simulink model "uz_ParameterID"  (R2021a)
settings: Solver=FixedStepDiscrete  StartTime=0.0  StopTime=160  FixedStep=0.000005  RelTol=1e-3  EnableMultiTasking=on
model workspace (MATLAB code in the model file):
  | cmdLim = Simulink.Parameter;
  | cmdLim.Value = 15;
  | cmdLim.Description = 'Limit for controlling the maximum surface command angle.';
  | cmdLim.Min = 0;
  | cmdLim.Max = 90;
  | cmdLim.DocUnits = 'deg';
  | 
  | dispGain = Simulink.Parameter;
  | dispGain.Value = 0.75;
  | dispGain.Description = 'Gain applied to the displacement error.';
  | dispGain.Min = 0;
  | dispGain.Max = [];
  | dispGain.DocUnits = 'deg/sec/deg';
  | 
  | dispLim = Simulink.Parameter;
  | dispLim.Value = 30;
  | dispLim.Description = 'Limit for controlling the maximum commanded angle.';
  | dispLim.Min = 0;
  | dispLim.Max = 180;
  | dispLim.DocUnits = 'deg';
  | 
  | intGain = Simulink.Parameter;
  | intGain.Value = 0.5;
  | intGain.Description = 'Gain applied to the integral error.';
  | intGain.Min = 0;
  | intGain.Max = [];
  | intGain.DocUnits = 'deg/sec/deg/sec';
  | 
  | intLim = Simulink.Parameter;
  | intLim.Value = 5;
  | intLim.Description = 'Limit for controlling the maximum commanded angle.';
  | intLim.Min = 0;
  | intLim.Max = 90;
  | intLim.DocUnits = 'deg';
  | 
  | rateGain = Simulink.Parameter;
  | rateGain.Value = 2;
  | rateGain.Description = 'Gain applied to the rate error.';
  | rateGain.Min = 0;
  | rateGain.Max = [];
  | rateGain.DocUnits = 'deg/deg/sec';
  | 
  | rateLim = Simulink.Parameter;
  | rateLim.Value = 6;
  | rateLim.Description = 'Limit for controlling the maximum commanded angle.';
  | rateLim.Min = 0;
  | rateLim.Max = 180;
  | rateLim.DocUnits = 'deg/sec';
  | 
  | hdgGain = Simulink.Parameter;
  | hdgGain.Value = 0.015;
values from neighbouring files (symbols this model uses):
  d_d_TMS = 0.005    [Parameter_Init_Buehler_201.m]
  d_f_hardware = 200000    [Parameter_Init_Buehler_201.m]
  d_f_states = 20000    [Parameter_Init_Buehler_201.m]
  d_i_max = 15    [Parameter_Init_Buehler_201.m]
  d_i_min = -d_i_max    (= -15)    [Parameter_Init_Buehler_201.m]
  d_I_n = 8    [Parameter_Init_Buehler_201.m]
  d_J_Coupling_M_E = 2e-6    (= 2e-06)    [Parameter_Init_Buehler_201.m]
  d_J_Coupling_M_Ms = 2e-20    [Parameter_Init_Buehler_201.m]
  d_J_Ms_L = d_J_Ms_M    (= 1.26363648e-05)    [Parameter_Init_Buehler_201.m]
  d_J_Ms_M = 0.5*0.5*((0.5*d_d_Ms)^4)*3.14*d_l_Ms*d_rho_Ms    (= 1.26363648e-05)    [Parameter_Init_Buehler_201.m]
  d_Ki_id = 162.47    [Parameter_Init_Buehler_201.m]
  d_Ki_iq = 162.47    [Parameter_Init_Buehler_201.m]
  d_Ki_n = 1.982    [Parameter_Init_Buehler_201.m]
  d_Kp_id = 0.369    [Parameter_Init_Buehler_201.m]
  d_Kp_iq = 0.369    [Parameter_Init_Buehler_201.m]
  d_Kp_n = 0.198    [Parameter_Init_Buehler_201.m]
  d_L_d = 0.00031    [Parameter_Init_Buehler_201.m]
  d_L_q = 0.00033    [Parameter_Init_Buehler_201.m]
  d_n_n = 3200    [Parameter_Init_Buehler_201.m]
  d_p = 4    [Parameter_Init_Buehler_201.m]
  d_psi_pm = 0.0075    [Parameter_Init_Buehler_201.m]
  d_R_ph = d_R_ph_ph/2    (= 0.089)    [Parameter_Init_Buehler_201.m]
  d_y_max = 10    [Parameter_Init_Buehler_201.m]
  d_y_min = -d_y_max    (= -10)    [Parameter_Init_Buehler_201.m]
undefined symbols (not defined in the file or in its folder): i_dq, i_dq_ref, n_ref, V_abc, v_dq
libraries: fl_lib x47, nesl_utility x30, ee_lib x18, simulink x8, spsabctodq0Lib x2, spsdq0toabcLib x1, spsTriangleGeneratorLib x1
(part 4 of 4)

== system uz_ParameterID/Hardware/Switch f. TMS/closed ==
  Input : PMIOPort  Side=Left
  output : PMIOPort  Port=2  Side=Right
  connections:
  output/RConn1 -- Input/RConn1

== system uz_ParameterID/Hardware/Switch f. TMS/open ==
  Rotational Free End : fl_lib/Mechanical/Rotational Elements/Rotational Free End  w_specify=off  w_priority=None  w=0 rad/s  w_nominal_specify=off  w_nominal_unit=rad/s  w_nominal_value=1
      settings: SourceProductBaseCode=SS
  Rotational Free End1 : fl_lib/Mechanical/Rotational Elements/Rotational Free End  w_specify=off  w_priority=None  w=0 rad/s  w_nominal_specify=off  w_nominal_unit=rad/s  w_nominal_value=1
      settings: SourceProductBaseCode=SS
  Input : PMIOPort  Side=Left
  output : PMIOPort  Port=2  Side=Right
  connections:
  Rotational Free End1/LConn1 -- output/RConn1
  Input/RConn1 -- Rotational Free End/LConn1

== system uz_ParameterID/Hardware/coupling m. shaft/Inertia ==
  Trägheitsmoment3 : fl_lib/Mechanical/Rotational Elements/Inertia  Commented=on  inertia=d_J_Coupling_M_Ms kg*m^2  num_ports=foundation.enum.numPorts2.one  w_specify=off  w_priority=High  w=0 rad/s  w_nominal_specify=off  w_nominal_unit=rad/s  w_nominal_value=1  t_specify=off  t_priority=None  t=0 N*m  t_nominal_specify=off  t_nominal_unit=N*m  t_nominal_value=1
      settings: AttributesFormatString=J in [%<inertia_unit>]
  Input : PMIOPort  Side=Left
  output : PMIOPort  Port=2  Side=Right
  connections:
  Input/RConn1 -- Trägheitsmoment3/LConn1 -- output/RConn1

== system uz_ParameterID/Hardware/coupling m. shaft/Spring Damper System ==
  Rotational Spring : fl_lib/Mechanical/Rotational Elements/Rotational Spring  spr_rate=d_c_Coupling_M_Ms N*m/rad  w_specify=off  w_priority=None  w=0 rad/s  w_nominal_specify=off  w_nominal_unit=rad/s  w_nominal_value=1  t_specify=off  t_priority=None  t=0 N*m  t_nominal_specify=off  t_nominal_unit=N*m  t_nominal_value=1  phi_specify=off  phi_priority=High  phi=0 rad  phi_nominal_specify=off  phi_nominal_unit=rad  phi_nominal_value=1
  Trägheitsmoment1 : fl_lib/Mechanical/Rotational Elements/Inertia  inertia=d_J_Coupling_M_Ms/2 kg*m^2  num_ports=foundation.enum.numPorts2.one  w_specify=off  w_priority=High  w=0 rad/s  w_nominal_specify=off  w_nominal_unit=rad/s  w_nominal_value=1  t_specify=off  t_priority=None  t=0 N*m  t_nominal_specify=off  t_nominal_unit=N*m  t_nominal_value=1
      settings: AttributesFormatString=J in [%<inertia_unit>]
  Trägheitsmoment3 : fl_lib/Mechanical/Rotational Elements/Inertia  inertia=d_J_Coupling_M_Ms/2 kg*m^2  num_ports=foundation.enum.numPorts2.one  w_specify=off  w_priority=High  w=0 rad/s  w_nominal_specify=off  w_nominal_unit=rad/s  w_nominal_value=1  t_specify=off  t_priority=None  t=0 N*m  t_nominal_specify=off  t_nominal_unit=N*m  t_nominal_value=1
      settings: AttributesFormatString=J in [%<inertia_unit>]
  dm : fl_lib/Mechanical/Rotational Elements/Rotational Damper  Commented=on  D=0 N*m/(rad/s)  w_specify=off  w_priority=None  w=0 rad/s  w_nominal_specify=off  w_nominal_unit=rad/s  w_nominal_value=1  t_specify=off  t_priority=None  t=0 N*m  t_nominal_specify=off  t_nominal_unit=N*m  t_nominal_value=1
  Input : PMIOPort  Side=Left
  output : PMIOPort  Port=2  Side=Right
  connections:
  Rotational Spring/LConn1 -- dm/LConn1 -- Input/RConn1 -- Trägheitsmoment3/LConn1
  Trägheitsmoment1/LConn1 -- Rotational Spring/RConn1 -- dm/RConn1 -- output/RConn1

== system uz_ParameterID/FOC/uz_FOC_Current/id-PI-Controller with anti wind-up/Clamping circuit ==
  preSat : Inport  DisableCoverage=on  OutDataTypeStr=single
  preIntegrator : Inport  DisableCoverage=on  Port=2
  AND : Logic  DisableCoverage=on
  DataTypeConv1 : DataTypeConversion  DisableCoverage=on  OutDataTypeStr=int8  SaturateOnIntegerOverflow=on  RndMeth=Zero  LockScale=on
  DataTypeConv2 : DataTypeConversion  DisableCoverage=on  OutDataTypeStr=int8  SaturateOnIntegerOverflow=on  RndMeth=Zero  LockScale=on
  DeadZone : DeadZone  DisableCoverage=on  LowerValue=d_y_min  UpperValue=d_y_max  SaturateOnIntegerOverflow=on
  Equal : RelationalOperator  DisableCoverage=on  Operator===  RndMeth=Nearest  InputSameDT=on
  NotEqual : RelationalOperator  DisableCoverage=on  Operator=~=  RndMeth=Nearest  InputSameDT=on
  SignDeltaU : Signum  DisableCoverage=on
  SignPreIntegrator : Signum  DisableCoverage=on
  ZeroGain : Gain  DisableCoverage=on  Gain=0  ParamDataTypeStr=double  OutDataTypeStr=single  SaturateOnIntegerOverflow=on
  Clamp : Outport  DisableCoverage=on  VectorParamsAs1DForOutWhenUnconnected=off
  wires:
  preSat/1 -> ZeroGain/1, DeadZone/1
  preIntegrator/1 -> SignPreIntegrator/1
  ZeroGain/1 -> NotEqual/1
  DeadZone/1 -> NotEqual/2, SignDeltaU/1
  SignDeltaU/1 -> DataTypeConv1/1
  DataTypeConv1/1 -> Equal/1
  SignPreIntegrator/1 -> DataTypeConv2/1
  DataTypeConv2/1 -> Equal/2
  NotEqual/1 -> AND/1
  Equal/1 -> AND/2
  AND/1 -> Clamp/1

== system uz_ParameterID/FOC/uz_FOC_Current/iq-PI-Controller with anti wind-up/Clamping circuit ==
  preSat : Inport  DisableCoverage=on  OutDataTypeStr=single
  preIntegrator : Inport  DisableCoverage=on  Port=2
  AND : Logic  DisableCoverage=on
  DataTypeConv1 : DataTypeConversion  DisableCoverage=on  OutDataTypeStr=int8  SaturateOnIntegerOverflow=on  RndMeth=Zero  LockScale=on
  DataTypeConv2 : DataTypeConversion  DisableCoverage=on  OutDataTypeStr=int8  SaturateOnIntegerOverflow=on  RndMeth=Zero  LockScale=on
  DeadZone : DeadZone  DisableCoverage=on  LowerValue=d_y_min  UpperValue=d_y_max  SaturateOnIntegerOverflow=on
  Equal : RelationalOperator  DisableCoverage=on  Operator===  RndMeth=Nearest  InputSameDT=on
  NotEqual : RelationalOperator  DisableCoverage=on  Operator=~=  RndMeth=Nearest  InputSameDT=on
  SignDeltaU : Signum  DisableCoverage=on
  SignPreIntegrator : Signum  DisableCoverage=on
  ZeroGain : Gain  DisableCoverage=on  Gain=0  ParamDataTypeStr=double  OutDataTypeStr=single  SaturateOnIntegerOverflow=on
  Clamp : Outport  DisableCoverage=on  VectorParamsAs1DForOutWhenUnconnected=off
  wires:
  preSat/1 -> ZeroGain/1, DeadZone/1
  preIntegrator/1 -> SignPreIntegrator/1
  ZeroGain/1 -> NotEqual/1
  DeadZone/1 -> NotEqual/2, SignDeltaU/1
  SignDeltaU/1 -> DataTypeConv1/1
  DataTypeConv1/1 -> Equal/1
  SignPreIntegrator/1 -> DataTypeConv2/1
  DataTypeConv2/1 -> Equal/2
  NotEqual/1 -> AND/1
  Equal/1 -> AND/2
  AND/1 -> Clamp/1

== system uz_ParameterID/FOC/uz_FOC_Speed/omega-PI-Controller with anti wind-up/Clamping circuit ==
  preSat : Inport  DisableCoverage=on  OutDataTypeStr=single
  preIntegrator : Inport  DisableCoverage=on  Port=2
  AND : Logic  DisableCoverage=on
  DataTypeConv1 : DataTypeConversion  DisableCoverage=on  OutDataTypeStr=int8  SaturateOnIntegerOverflow=on  RndMeth=Zero  LockScale=on
  DataTypeConv2 : DataTypeConversion  DisableCoverage=on  OutDataTypeStr=int8  SaturateOnIntegerOverflow=on  RndMeth=Zero  LockScale=on
  DeadZone : DeadZone  DisableCoverage=on  LowerValue=d_i_min  UpperValue=d_i_max  SaturateOnIntegerOverflow=on
  Equal : RelationalOperator  DisableCoverage=on  Operator===  RndMeth=Nearest  InputSameDT=on
  NotEqual : RelationalOperator  DisableCoverage=on  Operator=~=  RndMeth=Nearest  InputSameDT=on
  SignDeltaU : Signum  DisableCoverage=on
  SignPreIntegrator : Signum  DisableCoverage=on
  ZeroGain : Gain  DisableCoverage=on  Gain=0  ParamDataTypeStr=double  OutDataTypeStr=single  SaturateOnIntegerOverflow=on
  Clamp : Outport  DisableCoverage=on  VectorParamsAs1DForOutWhenUnconnected=off
  wires:
  preSat/1 -> ZeroGain/1, DeadZone/1
  preIntegrator/1 -> SignPreIntegrator/1
  ZeroGain/1 -> NotEqual/1
  DeadZone/1 -> NotEqual/2, SignDeltaU/1
  SignDeltaU/1 -> DataTypeConv1/1
  DataTypeConv1/1 -> Equal/1
  SignPreIntegrator/1 -> DataTypeConv2/1
  DataTypeConv2/1 -> Equal/2
  NotEqual/1 -> AND/1
  Equal/1 -> AND/2
  AND/1 -> Clamp/1

== matlab function uz_ParameterID/Hardware/12bit ADC1 ==
  data: u input; y output
function y = fcn(u)
%#codegen

y = u*2048/5;

== matlab function uz_ParameterID/Hardware/12bit ADC ==
  data: u input; y output
function y = fcn(u)
%#codegen

y = u*2048/5;

== matlab function uz_ParameterID/Hardware/12bit ADC2 ==
  data: u input; y output
function y = fcn(u)
%#codegen

y = u*2048/5;

== matlab function uz_ParameterID/FOC/Busselector ==
  data: ControlFlags input Bus: uz_ParaID_ControlFlags_t; FOC_state_outputs output Bus: uz_ParaID_Controller_Parameters_output_t; ElectricalID_FOC_input input Bus: uz_ParaID_Controller_Parameters_output_t; FrictionID_FOC_input input Bus: uz_ParaID_Controller_Parameters_output_t; FluxMapID_FOC_input input Bus: uz_ParaID_Controller_Parameters_output_t; TwoMassID_FOC_input input Bus: uz_ParaID_Controller_Parameters_output_t; FOCControl_input input Bus: uz_ParaID_Controller_Parameters_output_t
function FOC_state_outputs = fcn(ControlFlags,ElectricalID_FOC_input,....
    FrictionID_FOC_input,FluxMapID_FOC_input,TwoMassID_FOC_input,FOCControl_input)

switch ControlFlags.transNr
    case 0
        if(ControlFlags.finished_all_Offline_states==1)
            FOC_state_outputs           = FOCControl_input;
        else
        FOC_state_outputs.i_dq_ref.d          = single(0);
        FOC_state_outputs.i_dq_ref.q          = single(0);
        FOC_state_outputs.i_dq_ref.zero       = single(0);
        FOC_state_outputs.activeState         = uint16(0);
        FOC_state_outputs.n_ref_FOC           = single(0);
        FOC_state_outputs.enableFOC_speed     = boolean(0);
        FOC_state_outputs.enableFOC_current   = boolean(0);
        FOC_state_outputs.resetIntegrator     = boolean(0);
        FOC_state_outputs.Kp_id_out           = single(0);
        FOC_state_outputs.Kp_iq_out           = single(0);
        FOC_state_outputs.Kp_n_out            = single(0);
        FOC_state_outputs.Ki_id_out           = single(0);
        FOC_state_outputs.Ki_iq_out           = single(0);
        FOC_state_outputs.Ki_n_out            = single(0);
        end
    case 1
        FOC_state_outputs           = ElectricalID_FOC_input;
    case 2
        FOC_state_outputs           = TwoMassID_FOC_input;
    case 3
        FOC_state_outputs           = FrictionID_FOC_input;
    case 4
        FOC_state_outputs           = FluxMapID_FOC_input;
    otherwise
        FOC_state_outputs.i_dq_ref.d          = single(0);
        FOC_state_outputs.i_dq_ref.q          = single(0);
        FOC_state_outputs.i_dq_ref.zero       = single(0);
        FOC_state_outputs.activeState         = uint16(0);
        FOC_state_outputs.n_ref_FOC           = single(0);
        FOC_state_outputs.enableFOC_speed     = boolean(0);
        FOC_state_outputs.enableFOC_current   = boolean(0);
        FOC_state_outputs.resetIntegrator     = boolean(0);
        FOC_state_outputs.Kp_id_out           = single(0);
        FOC_state_outputs.Kp_iq_out           = single(0);
        FOC_state_outputs.Kp_n_out            = single(0);
        FOC_state_outputs.Ki_id_out           = single(0);
        FOC_state_outputs.Ki_iq_out           = single(0);
        FOC_state_outputs.Ki_n_out            = single(0);
end
end

== stateflow chart uz_ParameterID/ControlState ==
  settings: updateMethod=DISCRETE  sampleTime=1/d_f_states
  note: ControlState
  state ControlState
    entry:
    during:
    GlobalConfig_out.Reset = GlobalConfig_in.Reset;
    GlobalConfig_out.ACCEPT = GlobalConfig_in.ACCEPT;
    GlobalConfig_out.enableParameterID = GlobalConfig_in.enableParameterID;
    GlobalConfig_out.ElectricalID = GlobalConfig_in.ElectricalID;
    GlobalConfig_out.FrictionID = GlobalConfig_in.FrictionID
    GlobalConfig_out.TwoMassID = GlobalConfig_in.TwoMassID;
    GlobalConfig_out.FluxMapID = GlobalConfig_in.FluxMapID;
    GlobalConfig_out.OnlineID = GlobalConfig_in.OnlineID;
    GlobalConfig_out.sampleTimeISR = GlobalConfig_in.sampleTimeISR;
    state decideMotorID
      entry:
      during:
      if (GlobalConfig_in.ACCEPT == 1)
      decideIDstates;
      end
      if(ControlFlags.finished_all_Offline_states == 1 && GlobalConfig_in.OnlineID==1 && enteredOnlineID==0)
      ControlFlags.enableOnlineID=boolean(1);
      elseif (ControlFlags.finished_all_Offline_states == 1 && GlobalConfig_in.OnlineID==0 && enteredOnlineID==1)
      ControlFlags.enableOnlineID=boolean(0);
      end
      exit:
    state activateFrictionID
      entry:
      ControlFlags.startFrictionID=boolean(1);
      during:
      exit:
    state activateFluxMapID
      entry:
      ControlFlags.startFluxMapID=boolean(1);
      during:
      exit:
    state activateTwoMassID
      entry:
      ControlFlags.startTwoMassID=boolean(1);
      during:
      exit:
    state activateElectricalID
      entry:
      ControlFlags.startElectricalID=boolean(1);
      during:
      exit:
    state duringElectricalID
      entry:
      ControlFlags.startElectricalID=boolean(0);
      during:
      GlobalConfig_out.PMSM_config.Ld_Henry=ElectricalID_output.PMSM_parameters.Ld_Henry;
      GlobalConfig_out.PMSM_config.Lq_Henry=ElectricalID_output.PMSM_parameters.Lq_Henry;
      GlobalConfig_out.PMSM_config.R_ph_Ohm=ElectricalID_output.PMSM_parameters.R_ph_Ohm;
      GlobalConfig_out.PMSM_config.Psi_PM_Vs=ElectricalID_output.PMSM_parameters.Psi_PM_Vs;
      GlobalConfig_out.PMSM_config.polePairs=ElectricalID_output.PMSM_parameters.polePairs;
      GlobalConfig_out.PMSM_config.J_kg_m_squared=....
      ElectricalID_output.PMSM_parameters.J_kg_m_squared;
      GlobalConfig_out.Kp_id=ElectricalID_FOC_output.Kp_id_out;
      GlobalConfig_out.Kp_iq=ElectricalID_FOC_output.Kp_iq_out;
      GlobalConfig_out.Kp_n=ElectricalID_FOC_output.Kp_n_out;
      GlobalConfig_out.Ki_id=ElectricalID_FOC_output.Ki_id_out;
      GlobalConfig_out.Ki_iq=ElectricalID_FOC_output.Ki_iq_out;
      GlobalConfig_out.Ki_n=ElectricalID_FOC_output.Ki_n_out;
      exit:
    state duringTwoMassID
      entry:
      ControlFlags.startTwoMassID=boolean(0);
      during:
      exit:
    state duringFrictionID
      entry:
      ControlFlags.startFrictionID=boolean(0);
      during:
      exit:
    state duringFluxMapID
      entry:
      ControlFlags.startFluxMapID=boolean(0);
      during:
      exit:
    state finishedFrictionID
      entry:
      finishedFrictionID_loc=uint16(2);
      during:
      exit:
      ControlFlags.transNr=uint16(0);
    state finishedFluxMapID
      entry:
      finishedFluxMapID_loc=uint16(2);
      during:
      exit:
      ControlFlags.transNr=uint16(0);
    state finishedTwoMassID
      entry:
      finishedTwoMassID_loc=uint16(2);
      during:
      exit:
      ControlFlags.transNr=uint16(0);
    state finishedElectricalID
      entry:
      finishedElectricalID_loc=uint16(2);
      during:
      exit:
      ControlFlags.transNr=uint16(0);
    (default) -> decideMotorID
    decideMotorID -> activateElectricalID [order 1] : [ControlFlags.transNr==1 && finishedElectricalID_loc==0]
    activateElectricalID -> decideMotorID [order 2] : [GlobalConfig_in.ElectricalID==0]
        | {ControlFlags.transNr = 0}
    duringElectricalID -> decideMotorID [order 2] : [GlobalConfig_in.ElectricalID==0]
        | {ControlFlags.transNr = 0}
    finishedElectricalID -> decideMotorID
    finishedTwoMassID -> decideMotorID
    decideMotorID -> activateTwoMassID [order 3] : [ControlFlags.transNr==2 && finishedTwoMassID_loc==0]
    activateTwoMassID -> decideMotorID [order 2] : [GlobalConfig_in.TwoMassID==0]
        | {ControlFlags.transNr = 0}
    duringTwoMassID -> decideMotorID [order 2] : [GlobalConfig_in.TwoMassID==0]
        | {ControlFlags.transNr = 0}
    finishedFrictionID -> decideMotorID
    decideMotorID -> activateFrictionID [order 4] : [ControlFlags.transNr==3 && finishedFrictionID_loc==0]
    activateFrictionID -> decideMotorID [order 2] : [GlobalConfig_in.FrictionID==0]
        | {ControlFlags.transNr = 0}
    duringFrictionID -> decideMotorID [order 2] : [GlobalConfig_in.FrictionID==0]
        | {ControlFlags.transNr = 0}
    finishedFluxMapID -> decideMotorID
    decideMotorID -> activateFluxMapID [order 2] : [ControlFlags.transNr==4 && finishedFluxMapID_loc==0]
    activateFluxMapID -> decideMotorID [order 2] : [GlobalConfig_in.FluxMapID==0]
        | {ControlFlags.transNr = 0}
    duringFluxMapID -> decideMotorID [order 2] : [GlobalConfig_in.FluxMapID==0]
        | {ControlFlags.transNr = 0}
    activateElectricalID -> duringElectricalID [order 1] : [enteredElectricalID==1]
    activateTwoMassID -> duringTwoMassID [order 1] : [enteredTwoMassID==1]
    activateFrictionID -> duringFrictionID [order 1] : [enteredFrictionID==1]
    activateFluxMapID -> duringFluxMapID [order 1] : [enteredFluxMapID==1]
    duringTwoMassID -> finishedTwoMassID [order 1] : [finishedTwoMassID==1]
    duringFrictionID -> finishedFrictionID [order 1] : [finishedFrictionID==1]
    duringFluxMapID -> finishedFluxMapID [order 1] : [finishedFluxMapID==1]
    duringElectricalID -> finishedElectricalID [order 1] : [finishedElectricalID==1]
  state Waiting
    entry:
    initParams;
    %wait for activation of
    %FrictionID
    %donothing
  note: ---
  Waiting -> ControlState [order 1] : [GlobalConfig_in.enableParameterID==1 && ....
      | GlobalConfig_in.Reset==0]
  (default) -> Waiting
  ControlState -> Waiting : [GlobalConfig_in.Reset==1 ||....
      |  GlobalConfig_in.enableParameterID==0]
  Waiting -> Waiting [order 2] : [GlobalConfig_in.Reset==1]
  data: finishedFrictionID input boolean; finishedElectricalID input boolean; finishedTwoMassID input boolean; finishedFluxMapID input boolean; enteredFrictionID input boolean; enteredFluxMapID input boolean; enteredTwoMassID input boolean; enteredElectricalID input boolean; ElectricalID_output input Bus: uz_ParaID_ElectricalID_output_t; finishedElectricalID_loc local; finishedFrictionID_loc local; finishedTwoMassID_loc local; finishedFluxMapID_loc local; ElectricalID_FOC_output input Bus: uz_ParaID_Controller_Parameters_output_t; GlobalConfig_in input Bus: uz_ParaID_GlobalConfig_t; GlobalConfig_out output Bus: uz_ParaID_GlobalConfig_t; ControlFlags output Bus: uz_ParaID_ControlFlags_t; enteredOnlineID input
  function decideIDstates:
    | function decideIDstates
    | %If the specific Identification Part is not selected (==0), treat it, as if
    | %it has finished
    | if(GlobalConfig_in.ElectricalID==0)
    |     finishedElectricalID_loc=uint16(1);
    | elseif(finishedElectricalID==1)
    |     finishedElectricalID_loc=uint16(2);
    | end
    | 
    | if(GlobalConfig_in.FrictionID==0)
    |     finishedFrictionID_loc=uint16(1);
    | elseif(finishedFrictionID==1)
    |      finishedFrictionID_loc=uint16(2);
    | end
    | 
    | if(GlobalConfig_in.TwoMassID==0)
    |     finishedTwoMassID_loc=uint16(1);
    | elseif(finishedTwoMassID==1)
    |     finishedTwoMassID_loc=uint16(2);
    | end
    | 
    | if(GlobalConfig_in.FluxMapID==0)
    |     finishedFluxMapID_loc=uint16(1);
    | elseif(finishedFluxMapID==1)
    |     finishedFluxMapID_loc=uint16(2);    
    | end
    | 
    | if(ControlFlags.finished_all_Offline_states == 0)
    |     %Determine path through the ElectricalID-Stateflows
    |     if(GlobalConfig_in.ElectricalID==1 && enteredElectricalID==0 && finishedElectricalID_loc~=2 && finishedElectricalID==0)
    |             ControlFlags.transNr=uint16(1);
    |             finishedElectricalID_loc = uint16(0);
    |     end
    | 
    |     %Determine path through the TwoMassID-Stateflows
    |     if(GlobalConfig_in.TwoMassID==1 && enteredTwoMassID==0 && finishedElectricalID_loc~=0 && finishedTwoMassID_loc~=2 && finishedTwoMassID==0)
    |             ControlFlags.transNr=uint16(2);
    |             finishedTwoMassID_loc = uint16(0);
    |     end
    |     
    |     %Determine path through the FrictionID-Stateflows
    |     if(GlobalConfig_in.FrictionID==1 && enteredFrictionID==0 && finishedElectricalID_loc~=0....
    |        && finishedTwoMassID_loc~=0 && finishedFrictionID_loc~=2 && finishedFrictionID==0)
    |            ControlFlags.transNr=uint16(3);
    |            finishedFrictionID_loc = uint16(0);
    |     end
    | 
    |     %Determine path through the FluxMapID-Stateflows
    |     if(GlobalConfig_in.FluxMapID==1 && enteredFluxMapID==0 && finishedElectricalID_loc~=0....
    |       && finishedTwoMassID_loc~=0 && finishedFrictionID_loc~=0 && finishedFluxMapID_loc~=2 && finishedFluxMapID==0)
    |             ControlFlags.transNr=uint16(4);
    |             finishedFluxMapID_loc = uint16(0);
    |     end
    | end
    | 
    | if(finishedElectricalID_loc~=0 && finishedTwoMassID_loc~=0 && ....
    |         finishedFrictionID_loc~=0 && finishedFluxMapID_loc~=0)
    |     ControlFlags.finished_all_Offline_states = boolean(1);
    | end
    | 
    | end
  function initParams:
    | function initParams
    | %Initialize Variables
    | finishedElectricalID_loc=uint16(0);
    | finishedFrictionID_loc=uint16(0);
    | finishedTwoMassID_loc=uint16(0);
    | finishedFluxMapID_loc=uint16(0);
    | 
    | %Initialize Outputs
    | ControlFlags.startFrictionID             = boolean(0);
    | ControlFlags.startElectricalID           = boolean(0);
    | ControlFlags.startTwoMassID              = boolean(0);
    | ControlFlags.startFluxMapID              = boolean(0);
    | GlobalConfig_out                         = GlobalConfig_in;
    | ControlFlags.enableOnlineID              = boolean(0);
    | ControlFlags.transNr                     = uint16(0);
    | ControlFlags.finished_all_Offline_states = boolean(0);
    | end

== matlab function uz_ParameterID/InterpMeshGrid ==
  data: FluxMapData output Bus: uz_ParaID_FluxMapsData_t; psi_array_in input; i_rat input; OnlineID_input input
function FluxMapData = fcn(psi_array_in,i_rat,OnlineID_input)
%Author Philipp Gebhardt
% Oktober 2019

%This function is calculating the regular flux maps out of the irregular scatter data array stored in psi_array_in. The Outputs rangeX are containg the flux maps axis information which range is related to 3 times i_rat input.
%Furthermore the temperature dependency of the permanent flux is calculated if there are enough measuring values stored in the delta_psi_array. The temperature constant as well as the estimated error of permanent flux
%at reference temperature are given out on psi_temp_const and psi_temp_error outputs.  Using this temperature dependency the flux maps are updated with the permanent flux offset caused by the temperature which is given
%in on OnlineID_input.Wtemp input. 

%-----------------------------------------------------------------------------------------------------------------------------------------
%initalising Outputs
%-----------------------------------------------------------------------------------------------------------------------------------------

psi_array=zeros(6,100);
psi_array=psi_array_in;
delta_psi=zeros(100,1);

FluxMapData.psid_grid=single(zeros(20,20));
FluxMapData.psiq_grid=single(zeros(20,20));
FluxMapData.id_grid=single(zeros(20,20));
FluxMapData.iq_grid=single(zeros(20,20));
FluxMapData.range_id_Y=single(zeros(1,20));
FluxMapData.range_psid_Y=single(zeros(1,20));
FluxMapData.range_psiq_Y=single(zeros(1,20));
FluxMapData.range_psid_X=single(zeros(1,20));
FluxMapData.range_psiq_X=single(zeros(1,20));
FluxMapData.range_iq_Y=single(zeros(1,20));
FluxMapData.range_iq_X=single(zeros(1,20));
FluxMapData.range_id_X=single(zeros(1,20));
FluxMapData.psi_temp_const=single(0.000001);
FluxMapData.psi_temp_error=single(0);



range_psid_X_in=single(zeros(1,20));
range_psid_Y_in=single(zeros(1,20));
range_psiq_X_in=single(zeros(1,20));
range_psiq_Y_in=single(zeros(1,20));
range_id_X_in=single(zeros(1,20));
range_id_Y_in=single(zeros(1,20));
range_iq_X_in=single(zeros(1,20));
range_iq_Y_in=single(zeros(1,20));


%initalise range of flux maps axis
for t=single(0):single(19)
   range_psid_X_in(t+1)=-3*i_rat+t*4*i_rat/19;
   range_psid_Y_in(t+1)=-3*i_rat+t*6*i_rat/19;
   range_psiq_X_in(t+1)=-3*i_rat+t*4*i_rat/19;
   range_psiq_Y_in(t+1)=-3*i_rat+t*6*i_rat/19;
end

%Calculate flux deviation from amout of measuring values and counter sum,
%to average a big amount of measuring values 

for t=single(1):single(100)
    if (OnlineID_input.delta_psi(t,2)>5)
    delta_psi(t,1)=OnlineID_input.delta_psi(t,1)/OnlineID_input.delta_psi(t,2);
    end
end

%Calculate temperature constant with a regressionline, set second input "1"
%to resist outliers greater than 30% (relative to their neighbours)

[psi_temp_const_test,FluxMapData.psi_temp_error]=regressionline(delta_psi,1);

%check plausibility
if(psi_temp_const_test>0&&FluxMapData.psi_temp_const<10)%in mVs/°C
FluxMapData.psi_temp_const=psi_temp_const_test;
end


%correct temperature offset
 for k=single(1):single(100)
   if(psi_array(3,k)~=0)
    psi_array(5,k)=psi_array(5,k)+(psi_array(4,k)-OnlineID_input.Wtemp)*FluxMapData.psi_temp_const;
    psi_array(4,k)=OnlineID_input.Wtemp;
   end
end





%Inter- and extrapolation of the flux maps 
[FluxMapData.range_psid_X,FluxMapData.range_psid_Y,FluxMapData.psid_grid] = interpol_flux_scatter_psid ([psi_array(1,:);psi_array(2,:);psi_array(5,:);zeros(length(psi_array(1,:)))],range_psid_X_in,range_psid_Y_in);
[FluxMapData.range_psiq_X,FluxMapData.range_psiq_Y,FluxMapData.psiq_grid] = interpol_flux_scatter_psiq ([psi_array(1,:);psi_array(2,:);psi_array(6,:);zeros(length(psi_array(1,:)))],range_psiq_X_in,range_psiq_Y_in);

%initialise range of inverse flux maps axis
for t=single(0):single(19)
   range_id_X_in(t+1)=min(min(FluxMapData.psid_grid))+t*(max(max(FluxMapData.psid_grid))-min(min(FluxMapData.psid_grid)))/19;
   range_id_Y_in(t+1)=min(min(FluxMapData.psiq_grid))+t*(max(max(FluxMapData.psiq_grid))-min(min(FluxMapData.psiq_grid)))/19;
   range_iq_X_in(t+1)=min(min(FluxMapData.psid_grid))+t*(max(max(FluxMapData.psid_grid))-min(min(FluxMapData.psid_grid)))/19;
   range_iq_Y_in(t+1)=min(min(FluxMapData.psiq_grid))+t*(max(max(FluxMapData.psiq_grid))-min(min(FluxMapData.psiq_grid)))/19;
end

%Inter and extrapolate inverse flux maps
[FluxMapData.range_id_X,FluxMapData.range_id_Y,FluxMapData.id_grid] = interpol_flux_scatter_psid ([psi_array(5,:);psi_array(6,:);psi_array(1,:);zeros(length(psi_array(1,:)))],range_id_X_in,range_id_Y_in);
[FluxMapData.range_iq_X,FluxMapData.range_iq_Y,FluxMapData.iq_grid] = interpol_flux_scatter_psiq ([psi_array(5,:);psi_array(6,:);psi_array(2,:);zeros(length(psi_array(1,:)))],range_iq_X_in,range_iq_Y_in);

end

== stateflow chart uz_ParameterID/AutoRefCurrents ==
  settings: updateMethod=DISCRETE  sampleTime=1/d_f_states
  note: Philipp Gebhardt, October2019:
      |
      | Description of Control Reference Stateflow:
      |
      | This Stateflow chart is used to generate an cyclic current reference input of d- and q- current. The combinations are circularly arranged in the radius of imax_in.
      | The inputs niq and nid are the amount of measuring values in q- and d-current axis. The input speed_in is used to automatically control the sign of q-current to avoid
      | regenerative current feedback into the inverter.
  state waitState
    entry:
    %do nothing
    %wait for start
  state superstate
    entry:
    counter=single(19998);
    %counter=single(17498);
    iqcount=single(0);
    idcount=single(-AutoRefCurrentsConfig.id_points/3);
    AutoRefCurrents_output.i_dq_ref.d=single(0);
    AutoRefCurrents_output.i_dq_ref.q=single(0);
    imax=single(0);
    state stepstate
      entry:
      if(ActualValues.omega_m>0)
      imax=abs(AutoRefCurrentsConfig.max_current);
      end
      if(ActualValues.omega_m<0)
      imax=abs(AutoRefCurrentsConfig.max_current)*-1;
      end
      if((AutoRefCurrents_output.i_dq_ref.d*AutoRefCurrents_output.i_dq_ref.d+(imax*iqcount/AutoRefCurrentsConfig.iq_points)^2)^0.5<abs(imax))
      AutoRefCurrents_output.i_dq_ref.q=imax*iqcount/AutoRefCurrentsConfig.iq_points;
      else
      iqcount=single(1);
      AutoRefCurrents_output.i_dq_ref.q=imax*iqcount/AutoRefCurrentsConfig.iq_points;
      end
      if((AutoRefCurrents_output.i_dq_ref.q*AutoRefCurrents_output.i_dq_ref.q+(imax*idcount/AutoRefCurrentsConfig.id_points)^2)^0.5<abs(imax))
      AutoRefCurrents_output.i_dq_ref.d=-1*abs(imax)*idcount/AutoRefCurrentsConfig.id_points;
      else
      idcount=single(-AutoRefCurrentsConfig.id_points/3);
      AutoRefCurrents_output.i_dq_ref.d=-1*abs(imax)*idcount/AutoRefCurrentsConfig.id_points;
      end
      counter=single(0);
    state countstate
      entry:
      if(iqcount<AutoRefCurrentsConfig.iq_points)
      iqcount=iqcount+1;
      else
      iqcount=single(0);
      end
      if(idcount<AutoRefCurrentsConfig.id_points)
      idcount=idcount+1;
      else
      idcount=single(-AutoRefCurrentsConfig.id_points/3);
      end
      during:
      counter=counter+1;
    (default) -> countstate
    countstate -> stepstate : [counter==(2.0/GlobalConfig.sampleTimeISR)]
    stepstate -> countstate : [counter==0]
  (default) -> waitState
  waitState -> superstate : [AutoRefCurrentsConfig.enableCRS==1 &&....
      | AutoRefCurrentsConfig.Reset==0 &&....
      |  GlobalConfig.Reset==0 && GlobalConfig.ACCEPT==1&& ....
      | ControlFlags.finished_all_Offline_states==1]
  superstate -> waitState : [AutoRefCurrentsConfig.enableCRS==0 ||....
      |  AutoRefCurrentsConfig.Reset == 1 ||....
      | GlobalConfig.Reset==1]
      | {AutoRefCurrents_output.i_dq_ref.d=single(0);
      | AutoRefCurrents_output.i_dq_ref.q=single(0)}
  data: iqcount local; idcount local; counter local; ActualValues input Bus: uz_ParaID_ActualValues_t; imax local; GlobalConfig input Bus: uz_ParaID_GlobalConfig_t; AutoRefCurrentsConfig input Bus: uz_ParaID_AutoRefCurrentsConfig_t; AutoRefCurrents_output output Bus: uz_ParaID_AutoRefCurrents_output_t; ControlFlags input Bus: uz_ParaID_ControlFlags_t

== stateflow chart uz_ParameterID/FOC_ControlState ==
  settings: updateMethod=DISCRETE  sampleTime=1/d_f_states
  note: Control-States
  state FOC_ControlState
    entry:
    FOCControl_output.activeState = uint16(600);
    initParams;
    during:
    note: FOC current control
    state FOCcurrentControl 	%state 140
      entry:
      FOCControl_output.activeState = uint16(610);
      FOCControl_output.enableFOC_current=boolean(1);
      counter = uint32(1);
      during:
      FOCControl_output.i_dq_ref.q=GlobalConfig.i_dq_ref.q;
      FOCControl_output.i_dq_ref.d=GlobalConfig.i_dq_ref.d+i_d_Online_ref;
      exit:
      counter = uint32(1);
      FOCControl_output.enableFOC_current=boolean(0);
    state FOCdecider
      entry:
    note: FOC speed control
    note: change speed with sinusoidal trajectory in 0.2 sec
    state FOCspeed_speedChange 	%state 13.0
      entry:
      FOCControl_output.activeState = uint16(620);
      FOCControl_output.enableFOC_speed=boolean(1);
      counter = uint32(1);
      during:
      FOCControl_output.i_dq_ref.d = i_d_Online_ref+GlobalConfig.i_dq_ref.d;
      n_filt = single((single(counter)*GlobalConfig.sampleTimeISR*5)-....
      1/(2*pi)*sin(2*pi*single(counter)*GlobalConfig.sampleTimeISR*5));
      FOCControl_output.n_ref_FOC=((GlobalConfig.n_ref-n_ref_old)*n_filt)+n_ref_old;
      counter = counter + 1;
      exit:
      counter = uint32(1);
    state FOCspeed_constantSpeed 		%state 13.1
      entry:
      FOCControl_output.activeState = uint16(621);
      n_ref_old = GlobalConfig.n_ref;
      during:
      FOCControl_output.n_ref_FOC=GlobalConfig.n_ref;
      FOCControl_output.i_dq_ref.d=GlobalConfig.i_dq_ref.d +i_d_Online_ref;
      exit:
      counter = uint32(1);
      FOCControl_output.enableFOC_speed=boolean(0);
      note: constant speed
    (default) -> FOCdecider
    FOCdecider -> FOCcurrentControl 	%state 140 [order 1] : [controlType==0]
    FOCdecider -> FOCspeed_speedChange 	%state 13.0 [order 2] : [controlType==1]
    FOCspeed_constantSpeed 		%state 13.1 -> FOCspeed_speedChange 	%state 13.0 : [GlobalConfig.n_ref~=n_ref_old]
    FOCspeed_speedChange 	%state 13.0 -> FOCspeed_constantSpeed 		%state 13.1 : after(0.2,sec)
  state Waiting
    entry:
    %wait for activation of
    %FOCcontrol
    %donothing
  note: ---
  Waiting -> FOC_ControlState : [GlobalConfig.Reset==0 && ControlFlags.finished_all_Offline_states==1]
  (default) -> Waiting
  FOC_ControlState -> Waiting : [GlobalConfig.Reset==1]
  data: n_ref_old local; n_filt local; i_d_R_online local; counter local; FOCControl_output output Bus: uz_ParaID_Controller_Parameters_output_t; J local; measArray1 local; d local; i_d_Online_ref input; GlobalConfig input Bus: uz_ParaID_GlobalConfig_t; ControlFlags input Bus: uz_ParaID_ControlFlags_t; controlType input
  function initParams:
    | function initParams
    | 
    | % initialize variables
    | n_filt              = single(0.0);
    | n_ref_old           = single(0.0);
    | counter 			= uint32(1);
    | measArray1			= single(zeros(1024,1));
    | i_d_R_online        = single(0.0);
    | d        			= single(zeros(2048,1));
    | J 					= single(zeros(2048,2));
    | 
    | %Outputs
    | FOCControl_output.Ki_n_out          = single(GlobalConfig.Ki_n);
    | FOCControl_output.Ki_iq_out         = single(GlobalConfig.Ki_iq);
    | FOCControl_output.Ki_id_out         = single(GlobalConfig.Ki_id);
    | FOCControl_output.Kp_n_out          = single(GlobalConfig.Kp_n);
    | FOCControl_output.Kp_iq_out         = single(GlobalConfig.Kp_iq);
    | FOCControl_output.Kp_id_out         = single(GlobalConfig.Kp_id);
    | FOCControl_output.n_ref_FOC         = single(0.0);
    | FOCControl_output.i_dq_ref.d        = single(0.0);
    | FOCControl_output.i_dq_ref.q        = single(0.0);
    | FOCControl_output.i_dq_ref.zero      = single(0.0);
    | FOCControl_output.enableFOC_speed   = boolean(0);
    | FOCControl_output.enableFOC_current	= boolean(0);
    | FOCControl_output.resetIntegrator   = boolean(0);
    | FOCControl_output.activeState       = uint16(0);
    | 
    | end

== matlab function uz_ParameterID/CleanPsiArray ==
  data: OnlineID_output input; psi_array_out output; eta_c input; array_cleaned_flag output boolean; n_flux_points output
function [psi_array_out,array_cleaned_flag,n_flux_points]=clean_psi_array(OnlineID_output,eta_c)
% Author Philipp Gebhardt
% Oktober 2019

%This function is cleaning the array storing the measurement values, which always consits of a d-q-current combination a winding temperature and a speed value such as a d-q-flux combination
%The function is searching for measuring pairs which are closer than eta_c to their neighbours. In this case it is averaging these similar pairs to avoid measuring values storing the same information. 
%This is essential for calculating a wide ranging flux maps out of this array.
%Furthermore there is an output n_flux_points giving back the amount of independent measuring pairs


%Initialising Outputs
n_flux_points=single(1);
psi_array_out=single(zeros(6,100));
clean_curr_count=single(0);
array_cleaned_flag=boolean(0);

if(OnlineID_output.clean_array == 1)
% Searching for similar Datapairs
for(k=single(1):single(length(OnlineID_output.psi_array(1,:))))
    eta_count=0;
   
    if (OnlineID_output.psi_array(3,k)~=0)
        for(t=single(1):single(length(OnlineID_output.psi_array(1,:))))
            if (OnlineID_output.psi_array(3,t)~=0)
                if(k<t)    
                    if( (    (OnlineID_output.psi_array(1,k)-OnlineID_output.psi_array(1,t))^2  +...
                        (OnlineID_output.psi_array(2,k)-OnlineID_output.psi_array(2,t))^2     )^0.5 < eta_c )       
        %Averaging Datapairs if they are to close to each other
        
                        OnlineID_output.psi_array(1,t)=(OnlineID_output.psi_array(1,k)+OnlineID_output.psi_array(1,t))*0.5;
                        OnlineID_output.psi_array(2,t)=(OnlineID_output.psi_array(2,k)+OnlineID_output.psi_array(2,t))*0.5;
                        OnlineID_output.psi_array(3,t)=(OnlineID_output.psi_array(3,k)+OnlineID_output.psi_array(3,t))*0.5;
                        OnlineID_output.psi_array(4,t)=(OnlineID_output.psi_array(4,k)+OnlineID_output.psi_array(4,t))*0.5;                    
                        OnlineID_output.psi_array(5,t)=(OnlineID_output.psi_array(5,k)+OnlineID_output.psi_array(5,t))*0.5;
                        OnlineID_output.psi_array(6,t)=(OnlineID_output.psi_array(6,k)+OnlineID_output.psi_array(6,t))*0.5;     
                        OnlineID_output.psi_array(1:6,k)=0;
                        eta_count=1;  
                    end    
                end
            end
     
            if eta_count==1
                break
            end     
        end 
            if(eta_count==0)       
                %Accept values if there is enough distance between them
                clean_curr_count=clean_curr_count+1;
                psi_array_out(1,clean_curr_count)=OnlineID_output.psi_array(1,k);
                psi_array_out(2,clean_curr_count)=OnlineID_output.psi_array(2,k);
                psi_array_out(3,clean_curr_count)=OnlineID_output.psi_array(3,k);
                psi_array_out(4,clean_curr_count)=OnlineID_output.psi_array(4,k);
                psi_array_out(5,clean_curr_count)=OnlineID_output.psi_array(5,k);
                psi_array_out(6,clean_curr_count)=OnlineID_output.psi_array(6,k);
            end
    end
end

% Count flux points
for(k=single(1):single(length(psi_array_out(1,:))))  
    if(psi_array_out(1,k)~=0||psi_array_out(2,k)~=0||psi_array_out(3,k)~=0)       
           n_flux_points=k;
    end    
end

array_cleaned_flag=boolean(1);
end
return;

== matlab function uz_ParameterID/dqTrans/VoltageTransformation/Filterkorrektur_Hardware ==
  data: phi output; u input; y output; omega input; phi input

function [phi,y]= fcn(u,omega, phi)

R=95300;%ohm
RL=8200;%ohm
C=0.000000047;%Farrad
T=(RL*R*C)/(R+RL);

 w=omega;
%Filter zur Kompensation des Phasenversatz der Spannungen
 for i=single(1):single(3)
     %Rückgängigkmachen der ADC Umrechung und umkehren der Filterfunktion
u(i)=u(i)*(1+( w*T)^2)^0.5;
 end
 

phi=(phi)- atan(  w*T   );%atan(  w*T   );%*(1.08);


y = u;

== matlab function uz_ParameterID/FOC/Space vector limitation ==
  data: v_d_limit output; v_q_limit output; ActualValues input; v_d_in input single; v_q_in input; limit_on output boolean
% Algorithm for voltage space vector limitation
% 
% Quelle:    Vector Control of Three-Phase AC Machines, S. 183
% Autoren:   Nguyen Phung Quang, Jörg-Andreas Dittrich
%            Springer, 2015,Second Edition


function [v_d_limit, v_q_limit,limit_on] = fcn(ActualValues,v_d_in, v_q_in)
% max amplitude of the space vectors
   % with addition of 3rd harmonics   U^_LN = V_DC/2;
   %V_DC_max = V_DC*0.5;
   %with offset addition of 3rd harmonics  V^_LN = V_DC/sqrt(3);
   V_SV_max =ActualValues.V_DC/sqrt(3);

% absolue value of the space vector from vd and vq
V_SV_abs = sqrt(v_d_in^2 + v_q_in^2);

% limitation necessary?
if ( V_SV_abs > V_SV_max )   
    limit_on = boolean(1);   % limitation is necessary -> generator or drive operation?
   
    if ((sign(ActualValues.omega_el)==sign(ActualValues.i_dq.q)) ) % drive operation      
        Error = 0;
        if ( (abs(v_d_in) > 0.95*V_SV_max) )
        %true
        v_d_limit = sign(v_d_in)*0.95*V_SV_max;
        v_q_limit = sign(v_q_in)*sqrt(V_SV_max^2-v_d_limit^2);
        Fall = 2;
        else
        %false
        v_d_limit = v_d_in;
        v_q_limit = sign(v_q_in)*sqrt(V_SV_max^2-v_d_limit^2);
        Fall = 1;
        end    
    
    
    elseif ((sign(ActualValues.omega_el)~=sign(ActualValues.i_dq.q)) ) % generator operation   
        Error = 0;
        if ( abs(v_q_in) > 0.95*V_SV_max )
        %true
        v_q_limit = sign(v_q_in)*0.95*V_SV_max;
        v_d_limit = sign(v_d_in)*sqrt(V_SV_max^2-v_q_limit^2);
        %v_d_limit = U_d;        Fall = 4;       
        else 
        % false
        v_q_limit = v_q_in;
        v_d_limit = sign(v_d_in)*sqrt(V_SV_max^2-v_q_limit^2);
        Fall = 3;
        end
        
    else % Error
    v_d_limit = v_d_in;
    v_q_limit = v_q_in;
    Error = 1;
    Fall = 5;
    end
    
else
% no limitation necessary
    v_d_limit = v_d_in;
    v_q_limit = v_q_in;
    limit_on = boolean(0);
    Error = 0;
    Fall = 0;
end

v_d_in = v_d_limit;
v_q_in = v_q_limit;
end

== matlab function uz_ParameterID/FOC/uz_FOC_Speed/Field Weakening/MATLAB Function ==
  data: I_max input single; id_soll output single; V_DC input single; R input single; Lq input single; Ld input single; psi_pm input single; omega_el input single; iq_max output; id_ref_input input
function [id_soll, iq_max]= field_weakening(I_max, V_DC, R, Lq, Ld, psi_pm, omega_el,id_ref_input)

%Maximum voltage vector
v_max_dq = single(0.95* V_DC/sqrt(single(3)));
fw_flag = boolean(0);
%Calculation of n_cut
a = single(I_max^2 * Lq^2 + psi_pm^2);
b = single(2*R*psi_pm*I_max);
c = single((I_max^2 * R^2)-v_max_dq^2);

omega_cut = single((-b + sqrt(b^2 - 4*a*c))/(2*a));


%Check if w_cut is valid
if omega_cut > 0 && isreal(single(omega_cut))  
    %Calcultation of Id_ref
    if omega_el > omega_cut
        fw_flag = boolean(1);
        id_ref_fw = single(psi_pm/Ld * (omega_cut/omega_el -1));
        if id_ref_fw < -I_max
            id_ref_fw = -I_max;
        end
    else
        id_ref_fw = single(0.0);
    end
else
    id_ref_fw = single(0.0);
end

if fw_flag == boolean(0)
    id_soll = single(id_ref_input);
elseif (fw_flag == boolean(1)) && (id_ref_input <= id_ref_fw)
    id_soll = single(id_ref_input);
else
    id_soll = single(id_ref_fw);
end

if id_soll < single(0.0)
   a_fw = single(R^2 + omega_el^2 * Lq^2);
   b_fw = single(2*R*omega_el*psi_pm);
   c_fw = single(id_soll^2 * R^2 -v_max_dq^2 + omega_el^2 * (psi_pm^2 + Ld^2 * id_soll^2 + 2*psi_pm*Ld*id_soll));
   
   iq_max = single((-b_fw + sqrt(b_fw^2 - 4*a_fw*c_fw))/(2*a_fw));
   if iq_max > single(sqrt(I_max^2 - id_soll^2))
      iq_max =  single(sqrt(I_max^2 - id_soll^2));
   end
else
    iq_max = single(sqrt(I_max^2 - id_soll^2));
end
